simulink model "Final_4"  (R2022b)
settings: Solver=ode45  StartTime=0.0  StopTime=20  MaxStep=0.1  RelTol=1e-3
libraries: simulink_extras x2, slpidlib x1, cstblocks x1
settings Model: Creator=asus  LastModifiedBy=asus

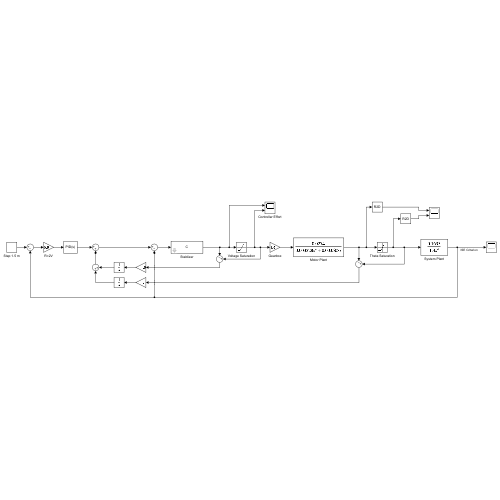
[thumbnail: Simulink's stored preview of the top-level diagram]
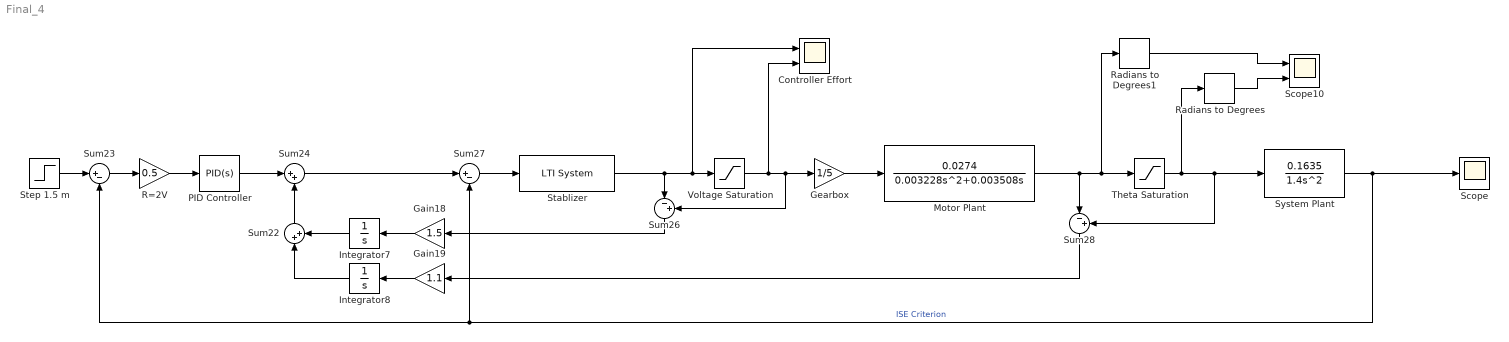
== system Final_4 ==
  Controller Effort : Scope  NumInputPorts=2
  Gain18 : Gain  Gain=1.5
  Gain19 : Gain  Gain=1.1
  Gearbox : Gain  Gain=1/5
  Integrator7 : Integrator
  Integrator8 : Integrator
  Motor Plant : TransferFcn  Numerator=[0.0274]  Denominator=[0.003228 0.003508 0]
  PID Controller : slpidlib/PID Controller  Controller=PID  Form=Parallel  TimeDomain=Continuous-time  UseExternalTs=off  SampleTime=-1  IntegratorMethod=Forward Euler  FilterMethod=Forward Euler  ControllerParametersSource=internal  P=2.927  I=2.2914  UseKiTs=off  D=0  N=100  UseFilter=on  TunerSelectOption=Transfer Function Based (PID Tuner App)  InitialConditionSource=internal  InitialConditionForIntegrator=0  InitialConditionForFilter=0  DifferentiatorICPrevScaledInput=0  ExternalReset=none  TrackingMode=off  Kt=1  LimitOutput=off  SatLimitsSource=internal  UpperSaturationLimit=inf  LowerSaturationLimit=-inf  LinearizeAsGain=on  AntiWindupMode=none  Kb=1  LimitIntegrator=off  UpperIntegratorSaturationLimit=inf  LowerIntegratorSaturationLimit=-inf  POutMin=[]  POutMax=[]  IOutMin=[]  IOutMax=[]  DOutMin=[]  DOutMax=[]  NOutMin=[]  NOutMax=[]  SumOutMin=[]  SumOutMax=[]  SaturationOutMin=[]  SaturationOutMax=[]  PParamMin=[]  PParamMax=[]  IParamMin=[]  IParamMax=[]  DParamMin=[]  DParamMax=[]  NParamMin=[]  NParamMax=[]  KbParamMin=[]  KbParamMax=[]  KtParamMin=[]  KtParamMax=[]  KbOutMin=[]  KbOutMax=[]  KtOutMin=[]  KtOutMax=[]  IntegratorOutMin=[]  IntegratorOutMax=[]  FilterOutMin=[]  FilterOutMax=[]  SumI1OutMin=[]  SumI1OutMax=[]  SumI2OutMin=[]  SumI2OutMax=[]  SumI3OutMin=[]  SumI3OutMax=[]  SumI4OutMin=[]  SumI4OutMax=[]  SumDOutMin=[]  SumDOutMax=[]  DifferentiatorOutMin=[]  DifferentiatorOutMax=[]  FilterDiffOutCoefMin=[]  FilterDiffOutCoefMax=[]  ReciprocalOutMin=[]  ReciprocalOutMax=[]  SumDenOutMin=[]  SumDenOutMax=[]  SumNumOutMin=[]  SumNumOutMax=[]  DivideOutMin=[]  DivideOutMax=[]  UdiffTsProdOutMin=[]  UdiffTsProdOutMax=[]  NTsProdOutMin=[]  NTsProdOutMax=[]  UintegralTsProdOutMin=[]  UintegralTsProdOutMax=[]  UngainTsProdOutMin=[]  UngainTsProdOutMax=[]  ClampingZeroOutDataTypeStr=Inherit: Inherit via back propagation  ClampingZeroOutMin=[]  ClampingZeroOutMax=[]  FilterDenConstantOutDataTypeStr=Inherit: Inherit via back propagation  FilterDenConstantOutMin=[]  FilterDenConstantOutMax=[]  PCopyOutDataTypeStr=Inherit: Inherit via back propagation  PCopyOutMin=[]  PCopyOutMax=[]  NCopyOutDataTypeStr=Inherit: Inherit via back propagation  NCopyOutMin=[]  NCopyOutMax=[]  IntegratorContinuousStateAttributes=''  IntegratorStateMustResolveToSignalObject=off  IntegratorRTWStateStorageClass=Auto  FilterContinuousStateAttributes=''  FilterStateMustResolveToSignalObject=off  FilterRTWStateStorageClass=Auto  ParallelPVariant=InternalParameters  IdealPVariant=Disabled  IVariant=InternalParameters  DVariant=InternalParameters  IntegratorVariant=Continuous  SatVariant=Disabled  AWVariant=Passthrough  PCopyVariant=Disabled  TRVariant=Disabled  FdbkBlocksVariant=Forward  IdealPFdbkVariant=Disabled  SatFdbkVariant=Disabled  DerivativeFilterVariant=ContFilter  NVariant=InternalParameters  NCopyVariant=Disabled  FilterICVariant=InternalICsFilter  IntegratorICVariant=InternalICs  ExternalResetVariant=Disabled  TRSumVariant=Passthrough  SumFdbkVariant=Disabled  SumVariant=Sum_PID  TsampFilterVariant=InternalTs  TsampNgainVariant=Passthrough  TsampIntegralVariant=Passthrough  ExternalSaturationOutDataTypeStr=Inherit: Same as second input
  R=2V : Gain  Gain=0.5
  Radians to Degrees : simulink_extras/Transformations/Radians to Degrees
  Radians to Degrees1 : simulink_extras/Transformations/Radians to Degrees
  Scope : Scope
  Scope10 : Scope  NumInputPorts=2
  Stablizer : cstblocks/LTI System  sys=C  IC=[]
  Step 1.5 m : Step  Time=0  After=1.5  SampleTime=0
  Sum22 : Sum  Inputs=|++
  Sum23 : Sum  Inputs=|+-
  Sum24 : Sum  Inputs=|++
  Sum26 : Sum  Inputs=|-+
  Sum27 : Sum  Inputs=|+-
  Sum28 : Sum  Inputs=|-+
  System Plant : TransferFcn  Numerator=[0.1635]  Denominator=[1.4 0 0]
  Theta Saturation : Saturate  UpperLimit=pi*0.49  LowerLimit=-pi*0.49
  Voltage Saturation : Saturate  UpperLimit=30  LowerLimit=-30
  wires:
  Sum27/1 -> Stablizer/1
  Integrator8/1 -> Sum22/1
  Step 1.5 m/1 -> Sum23/1
  Gain18/1 -> Integrator7/1
  Gearbox/1 -> Motor Plant/1
  Sum26/1 -> Gain18/1
  Sum24/1 -> Sum27/1
  Gain19/1 -> Integrator8/1
  System Plant/1 -> Scope/1, Sum23/2, Sum27/2  "ISE Criterion"
  Motor Plant/1 -> Radians to Degrees1/1, Theta Saturation/1, Sum28/1
  Sum28/1 -> Gain19/1
  Voltage Saturation/1 -> Sum26/2, Gearbox/1, Controller Effort/2
  Theta Saturation/1 -> System Plant/1, Sum28/2, Radians to Degrees/1
  Sum22/1 -> Sum24/2
  Stablizer/1 -> Controller Effort/1, Voltage Saturation/1, Sum26/1
  Integrator7/1 -> Sum22/2
  Radians to Degrees1/1 -> Scope10/1
  Radians to Degrees/1 -> Scope10/2
  Sum23/1 -> R=2V/1
  PID Controller/1 -> Sum24/1
  R=2V/1 -> PID Controller/1
